simulink model "SimpleSim"  (R2022b)
settings: Solver=VariableStepAuto  StartTime=0.0  StopTime=10.0  RelTol=1e-3
undefined symbols (not defined in the file or in its folder): environment, kite, winch
settings Model: Creator=jesse  LastModifiedBy=jesse
settings SolverCC: AlgebraicLoopSolver=TrustRegion
settings DebuggingCC: UnconnectedInputMsg=warning  UnconnectedOutputMsg=warning  UnconnectedLineMsg=warning  SFMachineParentedDataDiag=warning
settings ModelReferenceCC: EnableRefExpFcnMdlSchedulingChecks=on
settings RTWCC: DLArmComputeVersion=19.05

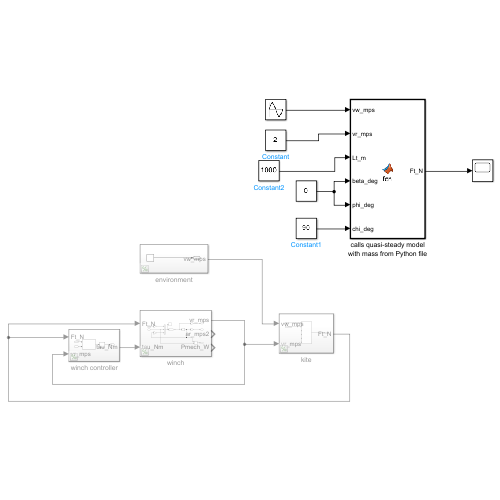
[thumbnail: Simulink's stored preview of the top-level diagram]
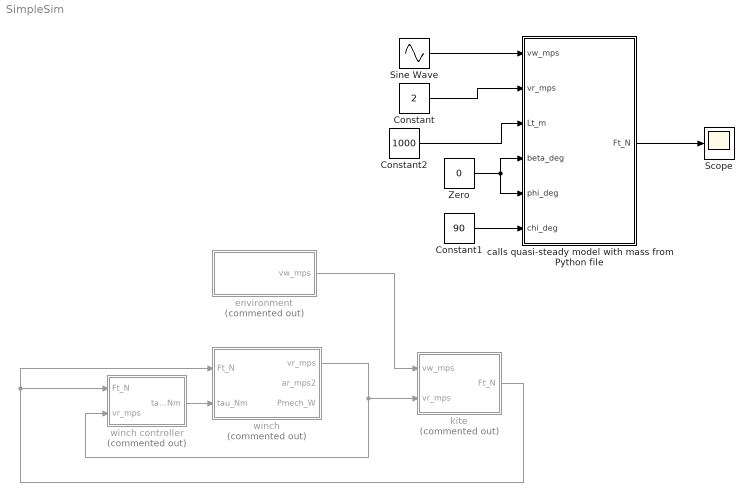
== system SimpleSim ==
  Constant : Constant  Value=2
  Constant1 : Constant  Value=90
  Constant2 : Constant  Value=1000
  Scope : Scope
  Sine Wave : Sin  Amplitude=10  Bias=10  SampleTime=0
  Zero : Constant  Value=0  OutDataTypeStr=Inherit: Inherit via back propagation
  calls quasi-steady model with mass from Python file : MATLAB Function  TreatAsAtomicUnit=on
  environment : Subsystem  Commented=on
  kite : Subsystem  Commented=on
  winch : Subsystem  Commented=on
  winch controller : Subsystem  Commented=on
  wires:
  winch/1(vr_mps) -> winch controller/2(vr_mps), kite/2(vr_mps)
  kite/1(Ft_N) -> winch/1(Ft_N), winch controller/1(Ft_N)
  winch controller/1(tau_Nm) -> winch/2(tau_Nm)
  environment/1(vw_mps) -> kite/1(vw_mps)
  calls quasi-steady model with mass from Python file/1(Ft_N) -> Scope/1
  Sine Wave/1 -> calls quasi-steady model with mass from Python file/1(vw_mps)
  Constant/1 -> calls quasi-steady model with mass from Python file/2(vr_mps)
  Zero/1 -> calls quasi-steady model with mass from Python file/5(phi_deg), calls quasi-steady model with mass from Python file/4(beta_deg)
  Constant1/1 -> calls quasi-steady model with mass from Python file/6(chi_deg)
  Constant2/1 -> calls quasi-steady model with mass from Python file/3(Lt_m)

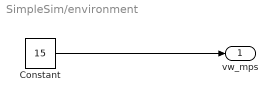
== system SimpleSim/environment ==
  Constant : Constant  Value=15
  vw_mps : Outport
  wires:
  Constant/1 -> vw_mps/1

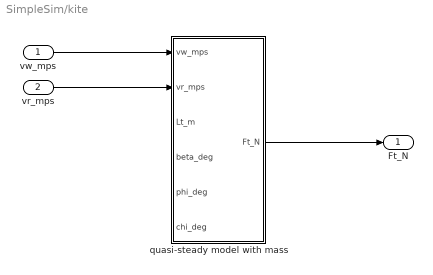
== system SimpleSim/kite ==
  vw_mps : Inport
  vr_mps : Inport  Port=2
  quasi-steady model with mass : Subsystem
  Ft_N : Outport
  wires:
  vw_mps/1 -> quasi-steady model with mass/1(vw_mps)
  vr_mps/1 -> quasi-steady model with mass/2(vr_mps)
  quasi-steady model with mass/1(Ft_N) -> Ft_N/1

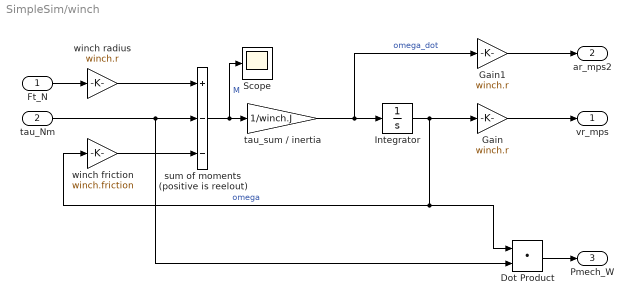
== system SimpleSim/winch ==
  Ft_N : Inport
  tau_Nm : Inport  Port=2
  Dot Product : DotProduct  OutDataTypeStr=Inherit: Inherit via internal rule
  Gain : Gain  Gain=winch.r
  Gain1 : Gain  Gain=winch.r
  Integrator : Integrator  InitialCondition=3.8
  Scope : Scope
  sum of moments (positive is reelout) : Sum  Inputs=+--
  tau_sum / inertia : Gain  Gain=1/winch.J
  winch friction : Gain  Gain=winch.friction
  winch radius : Gain  Gain=winch.r
  vr_mps : Outport
  ar_mps2 : Outport  Port=2
  Pmech_W : Outport  Port=3
  wires:
  Ft_N/1 -> winch radius/1
  winch friction/1 -> sum of moments (positive is reelout)/3
  sum of moments (positive is reelout)/1 -> Scope/1, tau_sum / inertia/1  "M"
  Dot Product/1 -> Pmech_W/1
  tau_sum / inertia/1 -> Gain1/1, Integrator/1  "omega_dot"
  tau_Nm/1 -> Dot Product/2, sum of moments (positive is reelout)/2
  winch radius/1 -> sum of moments (positive is reelout)/1
  Integrator/1 -> Gain/1, Dot Product/1, winch friction/1  "omega"
  Gain1/1 -> ar_mps2/1
  Gain/1 -> vr_mps/1

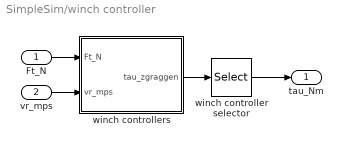
== system SimpleSim/winch controller ==
  Ft_N : Inport
  vr_mps : Inport  Port=2
  winch controller selector : Selector  InputPortWidth=3  IndexOptions=Index vector (dialog)  Indices=1  OutputSizes=1
  winch controllers : Subsystem
  tau_Nm : Outport
  wires:
  winch controller selector/1 -> tau_Nm/1
  winch controllers/1(tau_zgraggen) -> winch controller selector/1
  Ft_N/1 -> winch controllers/1(Ft_N)
  vr_mps/1 -> winch controllers/2(vr_mps)

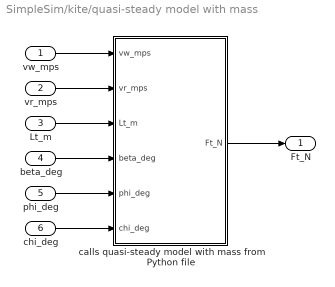
== system SimpleSim/kite/quasi-steady model with mass ==
  vw_mps : Inport
  vr_mps : Inport  Port=2
  Lt_m : Inport  Port=3
  beta_deg : Inport  Port=4
  phi_deg : Inport  Port=5
  chi_deg : Inport  Port=6
  calls quasi-steady model with mass from Python file : MATLAB Function  TreatAsAtomicUnit=on
  Ft_N : Outport
  wires:
  vw_mps/1 -> calls quasi-steady model with mass from Python file/1(vw_mps)
  vr_mps/1 -> calls quasi-steady model with mass from Python file/2(vr_mps)
  calls quasi-steady model with mass from Python file/1(Ft_N) -> Ft_N/1
  chi_deg/1 -> calls quasi-steady model with mass from Python file/6(chi_deg)
  phi_deg/1 -> calls quasi-steady model with mass from Python file/5(phi_deg)
  beta_deg/1 -> calls quasi-steady model with mass from Python file/4(beta_deg)
  Lt_m/1 -> calls quasi-steady model with mass from Python file/3(Lt_m)

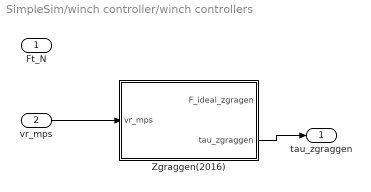
== system SimpleSim/winch controller/winch controllers ==
  Ft_N : Inport
  vr_mps : Inport  Port=2
  Zgraggen(2016) : MATLAB Function  TreatAsAtomicUnit=on
  tau_zgraggen : Outport
  wires:
  vr_mps/1 -> Zgraggen(2016)/1(vr_mps)
  Zgraggen(2016)/2(tau_zgraggen) -> tau_zgraggen/1

== matlab function SimpleSim/kite/quasi-steady model with mass/calls quasi-steady model with mass from Python file ==
  data: vw_mps input; Ft_N output; vr_mps input; Lt_m input; beta_deg input; phi_deg input; chi_deg input
function Ft_N = fcn(vw_mps, vr_mps, Lt_m, beta_deg, phi_deg, chi_deg)

Ft_N = pyrunfile("quasi_steady_model_for_Simulink.py", "Ft_N", ...
                 vw_mps=vw_mps, vr_mps=vr_mps,  Lt_m=Lt_m, ...
                 beta_deg=beta_deg, phi_deg=phi_deg, chi_deg=chi_deg);

end

== matlab function SimpleSim/winch controller/winch controllers/Zgraggen(2016) ==
  data: vr_mps input; F_ideal_zgragen output; environment parameter; tau_zgraggen output; winch parameter; kite parameter
function [F_ideal_zgragen, tau_zgraggen] = fcn(vr_mps, environment, winch, kite)

% Unpack parameters.
rho = environment.rho;
S = kite.S;
CL = kite.CL;
E = kite.E;
r = winch.r;

% Use calculation from Zgraggen:
% TODO: Zeta?
Zeta = 0.5 * rho * S * CL * E^2 * (1 + 1/E^2)^(3/2);
% TODO: This is only ideal for reeling factor 1/3. Which could be tuned
% further.
F_ideal_zgragen = 4*Zeta*vr_mps^2;

tau_zgraggen = F_ideal_zgragen*r;

== matlab function SimpleSim/calls quasi-steady model with mass from Python file ==
  data: vw_mps input; Ft_N output; vr_mps input; Lt_m input; beta_deg input; phi_deg input; chi_deg input
function Ft_N = fcn(vw_mps, vr_mps, Lt_m, beta_deg, phi_deg, chi_deg)

%     % From: https://nl.mathworks.com/matlabcentral/answers/359575-how-to-run-a-python-code-on-simulink
%     out = 0; % Has to be preassigned, otherwise Simulink throws an error
%     coder.extrinsic('py.Example.test') % Python functions have to be run extrinsically, meaning no C code generated
%     out = py.Example.test(1,3);
%     Ft_N = out;

%     Ft_N = 0;
%     coder.extrinsic('py.qsm_wrapper.calc_Ft') % Python functions have to be run extrinsically, meaning no C code generated
%     out = py.qsm_wrapper.calc_Ft(vw_mps, vr_mps, Lt_m, beta_deg, phi_deg, chi_deg);
%     Ft_N = out;

    Ft_N = 0;
    coder.extrinsic('py.qsm_wrapper2.calc_Ft') % Python functions have to be run extrinsically, meaning no C code generated
    out = py.qsm_wrapper2.calc_Ft(vw_mps, vr_mps, Lt_m, beta_deg, phi_deg, chi_deg);
    Ft_N = out;


%     Ft_N = 0; % Has to be preassigned, otherwise Simulink throws an error.
%     coder.extrinsic('py.Example.test2') % Python functions have to be run extrinsically, meaning no C code generated.
%     Ft_N = py.Example.test2(...
%     vw_mps,...
%     vr_mps,...
%     Lt_m,...
%     beta_deg,...
%     phi_deg,...
%     chi_deg);

end
